simulink model "LogSimulation"  (R2024a)
settings: Solver=FixedStepDiscrete  StartTime=0.0  StopTime=10.0  FixedStep=5e-5  RelTol=1e-3  EnableMultiTasking=on
settings Model: Creator=rdelpoux  LastModifiedBy=rdelpoux
settings DataIOCC: ExternalInput=dataLog.getElement('vdq'),dataLog.getElement('idq'),dataLog.getElement('omega')  LoadExternalInput=on

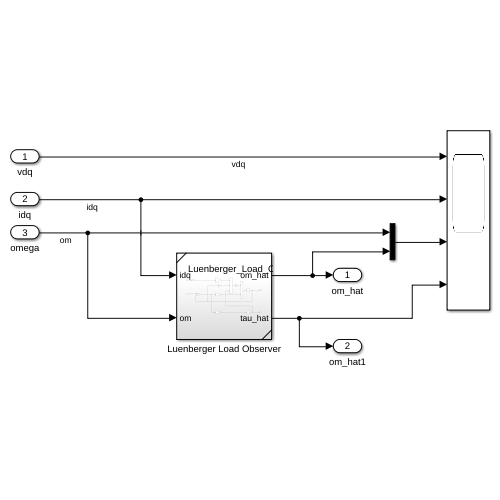
[thumbnail: Simulink's stored preview of the top-level diagram]
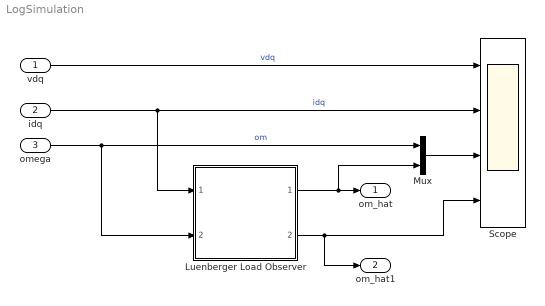
== system LogSimulation ==
  vdq : Inport  OutDataTypeStr=single  PortDimensions=2
  idq : Inport  Port=2  OutDataTypeStr=single  PortDimensions=2
  omega : Inport  Port=3  OutDataTypeStr=single  PortDimensions=1
  Luenberger Load Observer : Subsystem  ReferencedSubsystem=Luenberger_Load_Observer
  Mux : Mux  Inputs=2
  Scope : Scope  NumInputPorts=4
  om_hat : Outport
  om_hat1 : Outport  Port=2
  wires:
  vdq/1 -> Scope/1  "vdq"
  omega/1 -> Luenberger Load Observer/2, Mux/1  "om"
  idq/1 -> Luenberger Load Observer/1, Scope/2  "idq"
  Mux/1 -> Scope/3
  Luenberger Load Observer/2 -> om_hat1/1, Scope/4
  Luenberger Load Observer/1 -> om_hat/1, Mux/2
